simulink model "Pedal_Interpretation_exe"  (Simulink 7.0)
settings: Solver=ode4  StartTime=0.0  StopTime=88  FixedStep=0.01  RelTol=1e-3
InitFcn:
  | PedalInterp_para
values from neighbouring files (symbols this model uses):
  ped_min = 5    [PedalInterp_para.m]
  T_max_Brake = 4000    [PedalInterp_para.m]
  TI = 0    [PAS_callback.m]
undefined symbols (not defined in the file or in its folder): fzgbib, m_ab_100pro, m_ab_70pro, PedalInterpretation, v_bereich
libraries: simulink x320
(part 9 of 23)

== system Pedal_Interpretation_exe/TestData 1/SR-PI-02.2 Acceleration pedal interpretation/v = const & phi_Acc decreases & T_des_Drive < 0/Generate decrease 7/Generate  limited decrease for partition1 variant2 1 ==
  Repeating Sequence : Subsystem  mask(Repeating table){rep_seq_t=[0 T], rep_seq_y=[X0 XF]}
      mask prompts: rep_seq_t "Time values:"; rep_seq_y "Output values:"
      mask help: Output a repeating sequence of numbers specified in a table of time-value pairs. Values of time should be monotonically increasing.
      mask init: same as Pedal_Interpretation_exe/TestData 1/SR-PI-01.1 Brake Pedal recognition/phi_Brake < ped_min/Generate decrease 2/Generate  limited decrease for partition1 variant1 1/Repeating Sequence
      mask Help: Repeats cycle given in table. Time values should be monotonically increasing.
      mask Display: plot( disp_seq_t, disp_seq_y )
  Out1 : Outport  OutDataType=sfix(16)  OutScaling=2^0
  wires:
  Repeating Sequence/1(Out1) -> Out1/1

== system Pedal_Interpretation_exe/TestData 1/SR-PI-02.2 Acceleration pedal interpretation/v = const & phi_Acc decreases & T_des_Drive < 0/Generate decrease 7/TestDataVariants Sequence ==
  Constant : Constant  Value=2  OutDataType=sfix(16)  OutScaling=2^0
  Relational Operator : RelationalOperator  Operator=<=  LogicOutDataTypeMode=boolean
  Switch : Switch  Criteria=u2 ~= 0  OutDataType=sfix(16)  OutScaling=2^0
  Out1 : Outport  OutDataType=sfix(16)  OutScaling=2^0
  wires:
  [A] -> Relational Operator/1, Switch/1
  Constant/1 -> Relational Operator/2, Switch/3
  Relational Operator/1 -> Switch/2
  Switch/1 -> Out1/1

== system Pedal_Interpretation_exe/TestData 1/SR-PI-02.2 Acceleration pedal interpretation/v = const & phi_Acc decreases & T_des_Drive >= 0/Generate constant 6/Generate  constant for partition1 variant1 1 ==
  Repeating Sequence : Subsystem  mask(Repeating table){rep_seq_t=[0 T], rep_seq_y=[X0 X0]}
      mask prompts: rep_seq_t "Time values:"; rep_seq_y "Output values:"
      mask help: Output a repeating sequence of numbers specified in a table of time-value pairs. Values of time should be monotonically increasing.
      mask init: same as Pedal_Interpretation_exe/TestData 1/SR-PI-01.1 Brake Pedal recognition/phi_Brake < ped_min/Generate decrease 2/Generate  limited decrease for partition1 variant1 1/Repeating Sequence
      mask Help: Repeats cycle given in table. Time values should be monotonically increasing.
      mask Display: plot( disp_seq_t, disp_seq_y )
  Out1 : Outport  OutDataType=sfix(16)  OutScaling=2^0
  wires:
  Repeating Sequence/1(Out1) -> Out1/1

== system Pedal_Interpretation_exe/TestData 1/SR-PI-02.2 Acceleration pedal interpretation/v = const & phi_Acc decreases & T_des_Drive >= 0/Generate constant 6/Generate  constant for partition1 variant2 1 ==
  Repeating Sequence : Subsystem  mask(Repeating table){rep_seq_t=[0 T], rep_seq_y=[X0 X0]}
      mask prompts: rep_seq_t "Time values:"; rep_seq_y "Output values:"
      mask help: Output a repeating sequence of numbers specified in a table of time-value pairs. Values of time should be monotonically increasing.
      mask init: same as Pedal_Interpretation_exe/TestData 1/SR-PI-01.1 Brake Pedal recognition/phi_Brake < ped_min/Generate decrease 2/Generate  limited decrease for partition1 variant1 1/Repeating Sequence
      mask Help: Repeats cycle given in table. Time values should be monotonically increasing.
      mask Display: plot( disp_seq_t, disp_seq_y )
  Out1 : Outport  OutDataType=sfix(16)  OutScaling=2^0
  wires:
  Repeating Sequence/1(Out1) -> Out1/1

== system Pedal_Interpretation_exe/TestData 1/SR-PI-02.2 Acceleration pedal interpretation/v = const & phi_Acc decreases & T_des_Drive >= 0/Generate constant 6/Generate  constant for partition1 variant3 1 ==
  Repeating Sequence : Subsystem  mask(Repeating table){rep_seq_t=[0 T], rep_seq_y=[X0 X0]}
      mask prompts: rep_seq_t "Time values:"; rep_seq_y "Output values:"
      mask help: Output a repeating sequence of numbers specified in a table of time-value pairs. Values of time should be monotonically increasing.
      mask init: same as Pedal_Interpretation_exe/TestData 1/SR-PI-01.1 Brake Pedal recognition/phi_Brake < ped_min/Generate decrease 2/Generate  limited decrease for partition1 variant1 1/Repeating Sequence
      mask Help: Repeats cycle given in table. Time values should be monotonically increasing.
      mask Display: plot( disp_seq_t, disp_seq_y )
  Out1 : Outport  OutDataType=sfix(16)  OutScaling=2^0
  wires:
  Repeating Sequence/1(Out1) -> Out1/1

== system Pedal_Interpretation_exe/TestData 1/SR-PI-02.2 Acceleration pedal interpretation/v = const & phi_Acc decreases & T_des_Drive >= 0/Generate constant 6/Generate  constant for partition1 variant4 1 ==
  Repeating Sequence : Subsystem  mask(Repeating table){rep_seq_t=[0 T], rep_seq_y=[X0 X0]}
      mask prompts: rep_seq_t "Time values:"; rep_seq_y "Output values:"
      mask help: Output a repeating sequence of numbers specified in a table of time-value pairs. Values of time should be monotonically increasing.
      mask init: same as Pedal_Interpretation_exe/TestData 1/SR-PI-01.1 Brake Pedal recognition/phi_Brake < ped_min/Generate decrease 2/Generate  limited decrease for partition1 variant1 1/Repeating Sequence
      mask Help: Repeats cycle given in table. Time values should be monotonically increasing.
      mask Display: plot( disp_seq_t, disp_seq_y )
  Out1 : Outport  OutDataType=sfix(16)  OutScaling=2^0
  wires:
  Repeating Sequence/1(Out1) -> Out1/1

== system Pedal_Interpretation_exe/TestData 1/SR-PI-02.2 Acceleration pedal interpretation/v = const & phi_Acc decreases & T_des_Drive >= 0/Generate constant 6/Generate  constant for partition1 variant5 1 ==
  Repeating Sequence : Subsystem  mask(Repeating table){rep_seq_t=[0 T], rep_seq_y=[X0 X0]}
      mask prompts: rep_seq_t "Time values:"; rep_seq_y "Output values:"
      mask help: Output a repeating sequence of numbers specified in a table of time-value pairs. Values of time should be monotonically increasing.
      mask init: same as Pedal_Interpretation_exe/TestData 1/SR-PI-01.1 Brake Pedal recognition/phi_Brake < ped_min/Generate decrease 2/Generate  limited decrease for partition1 variant1 1/Repeating Sequence
      mask Help: Repeats cycle given in table. Time values should be monotonically increasing.
      mask Display: plot( disp_seq_t, disp_seq_y )
  Out1 : Outport  OutDataType=sfix(16)  OutScaling=2^0
  wires:
  Repeating Sequence/1(Out1) -> Out1/1

== system Pedal_Interpretation_exe/TestData 1/SR-PI-02.2 Acceleration pedal interpretation/v = const & phi_Acc decreases & T_des_Drive >= 0/Generate constant 6/TestDataVariants Sequence ==
  Constant : Constant  Value=5  OutDataType=sfix(16)  OutScaling=2^0
  Relational Operator : RelationalOperator  Operator=<=  LogicOutDataTypeMode=boolean
  Switch : Switch  Criteria=u2 ~= 0  OutDataType=sfix(16)  OutScaling=2^0
  Out1 : Outport  OutDataType=sfix(16)  OutScaling=2^0
  wires:
  [A] -> Relational Operator/1, Switch/1
  Constant/1 -> Relational Operator/2, Switch/3
  Relational Operator/1 -> Switch/2
  Switch/1 -> Out1/1

== system Pedal_Interpretation_exe/TestData 1/SR-PI-02.2 Acceleration pedal interpretation/v = const & phi_Acc decreases & T_des_Drive >= 0/Generate decrease 7/Generate  limited decrease for partition1 variant1 1 ==
  Repeating Sequence : Subsystem  mask(Repeating table){rep_seq_t=[0 T], rep_seq_y=[X0 XF]}
      mask prompts: rep_seq_t "Time values:"; rep_seq_y "Output values:"
      mask help: Output a repeating sequence of numbers specified in a table of time-value pairs. Values of time should be monotonically increasing.
      mask init: same as Pedal_Interpretation_exe/TestData 1/SR-PI-01.1 Brake Pedal recognition/phi_Brake < ped_min/Generate decrease 2/Generate  limited decrease for partition1 variant1 1/Repeating Sequence
      mask Help: Repeats cycle given in table. Time values should be monotonically increasing.
      mask Display: plot( disp_seq_t, disp_seq_y )
  Out1 : Outport  OutDataType=sfix(16)  OutScaling=2^0
  wires:
  Repeating Sequence/1(Out1) -> Out1/1

== system Pedal_Interpretation_exe/TestData 1/SR-PI-02.2 Acceleration pedal interpretation/v = const & phi_Acc decreases & T_des_Drive >= 0/Generate decrease 7/Generate  limited decrease for partition1 variant2 1 ==
  Repeating Sequence : Subsystem  mask(Repeating table){rep_seq_t=[0 T], rep_seq_y=[X0 XF]}
      mask prompts: rep_seq_t "Time values:"; rep_seq_y "Output values:"
      mask help: Output a repeating sequence of numbers specified in a table of time-value pairs. Values of time should be monotonically increasing.
      mask init: same as Pedal_Interpretation_exe/TestData 1/SR-PI-01.1 Brake Pedal recognition/phi_Brake < ped_min/Generate decrease 2/Generate  limited decrease for partition1 variant1 1/Repeating Sequence
      mask Help: Repeats cycle given in table. Time values should be monotonically increasing.
      mask Display: plot( disp_seq_t, disp_seq_y )
  Out1 : Outport  OutDataType=sfix(16)  OutScaling=2^0
  wires:
  Repeating Sequence/1(Out1) -> Out1/1

== system Pedal_Interpretation_exe/TestData 1/SR-PI-02.2 Acceleration pedal interpretation/v = const & phi_Acc decreases & T_des_Drive >= 0/Generate decrease 7/TestDataVariants Sequence ==
  Constant : Constant  Value=2  OutDataType=sfix(16)  OutScaling=2^0
  Relational Operator : RelationalOperator  Operator=<=  LogicOutDataTypeMode=boolean
  Switch : Switch  Criteria=u2 ~= 0  OutDataType=sfix(16)  OutScaling=2^0
  Out1 : Outport  OutDataType=sfix(16)  OutScaling=2^0
  wires:
  [A] -> Relational Operator/1, Switch/1
  Constant/1 -> Relational Operator/2, Switch/3
  Relational Operator/1 -> Switch/2
  Switch/1 -> Out1/1

== system Pedal_Interpretation_exe/TestData 1/SR-PI-02.2 Acceleration pedal interpretation/v = const & phi_Acc increases & T_des_Drive < 0/Generate constant 6/Generate  constant for partition1 variant1 1 ==
  Repeating Sequence : Subsystem  mask(Repeating table){rep_seq_t=[0 T], rep_seq_y=[X0 X0]}
      mask prompts: rep_seq_t "Time values:"; rep_seq_y "Output values:"
      mask help: Output a repeating sequence of numbers specified in a table of time-value pairs. Values of time should be monotonically increasing.
      mask init: same as Pedal_Interpretation_exe/TestData 1/SR-PI-01.1 Brake Pedal recognition/phi_Brake < ped_min/Generate decrease 2/Generate  limited decrease for partition1 variant1 1/Repeating Sequence
      mask Help: Repeats cycle given in table. Time values should be monotonically increasing.
      mask Display: plot( disp_seq_t, disp_seq_y )
  Out1 : Outport  OutDataType=sfix(16)  OutScaling=2^0
  wires:
  Repeating Sequence/1(Out1) -> Out1/1

== system Pedal_Interpretation_exe/TestData 1/SR-PI-02.2 Acceleration pedal interpretation/v = const & phi_Acc increases & T_des_Drive < 0/Generate constant 6/Generate  constant for partition1 variant2 1 ==
  Repeating Sequence : Subsystem  mask(Repeating table){rep_seq_t=[0 T], rep_seq_y=[X0 X0]}
      mask prompts: rep_seq_t "Time values:"; rep_seq_y "Output values:"
      mask help: Output a repeating sequence of numbers specified in a table of time-value pairs. Values of time should be monotonically increasing.
      mask init: same as Pedal_Interpretation_exe/TestData 1/SR-PI-01.1 Brake Pedal recognition/phi_Brake < ped_min/Generate decrease 2/Generate  limited decrease for partition1 variant1 1/Repeating Sequence
      mask Help: Repeats cycle given in table. Time values should be monotonically increasing.
      mask Display: plot( disp_seq_t, disp_seq_y )
  Out1 : Outport  OutDataType=sfix(16)  OutScaling=2^0
  wires:
  Repeating Sequence/1(Out1) -> Out1/1

== system Pedal_Interpretation_exe/TestData 1/SR-PI-02.2 Acceleration pedal interpretation/v = const & phi_Acc increases & T_des_Drive < 0/Generate constant 6/Generate  constant for partition1 variant3 1 ==
  Repeating Sequence : Subsystem  mask(Repeating table){rep_seq_t=[0 T], rep_seq_y=[X0 X0]}
      mask prompts: rep_seq_t "Time values:"; rep_seq_y "Output values:"
      mask help: Output a repeating sequence of numbers specified in a table of time-value pairs. Values of time should be monotonically increasing.
      mask init: same as Pedal_Interpretation_exe/TestData 1/SR-PI-01.1 Brake Pedal recognition/phi_Brake < ped_min/Generate decrease 2/Generate  limited decrease for partition1 variant1 1/Repeating Sequence
      mask Help: Repeats cycle given in table. Time values should be monotonically increasing.
      mask Display: plot( disp_seq_t, disp_seq_y )
  Out1 : Outport  OutDataType=sfix(16)  OutScaling=2^0
  wires:
  Repeating Sequence/1(Out1) -> Out1/1

== system Pedal_Interpretation_exe/TestData 1/SR-PI-02.2 Acceleration pedal interpretation/v = const & phi_Acc increases & T_des_Drive < 0/Generate constant 6/Generate  constant for partition1 variant4 1 ==
  Repeating Sequence : Subsystem  mask(Repeating table){rep_seq_t=[0 T], rep_seq_y=[X0 X0]}
      mask prompts: rep_seq_t "Time values:"; rep_seq_y "Output values:"
      mask help: Output a repeating sequence of numbers specified in a table of time-value pairs. Values of time should be monotonically increasing.
      mask init: same as Pedal_Interpretation_exe/TestData 1/SR-PI-01.1 Brake Pedal recognition/phi_Brake < ped_min/Generate decrease 2/Generate  limited decrease for partition1 variant1 1/Repeating Sequence
      mask Help: Repeats cycle given in table. Time values should be monotonically increasing.
      mask Display: plot( disp_seq_t, disp_seq_y )
  Out1 : Outport  OutDataType=sfix(16)  OutScaling=2^0
  wires:
  Repeating Sequence/1(Out1) -> Out1/1

== system Pedal_Interpretation_exe/TestData 1/SR-PI-02.2 Acceleration pedal interpretation/v = const & phi_Acc increases & T_des_Drive < 0/Generate constant 6/Generate  constant for partition1 variant5 1 ==
  Repeating Sequence : Subsystem  mask(Repeating table){rep_seq_t=[0 T], rep_seq_y=[X0 X0]}
      mask prompts: rep_seq_t "Time values:"; rep_seq_y "Output values:"
      mask help: Output a repeating sequence of numbers specified in a table of time-value pairs. Values of time should be monotonically increasing.
      mask init: same as Pedal_Interpretation_exe/TestData 1/SR-PI-01.1 Brake Pedal recognition/phi_Brake < ped_min/Generate decrease 2/Generate  limited decrease for partition1 variant1 1/Repeating Sequence
      mask Help: Repeats cycle given in table. Time values should be monotonically increasing.
      mask Display: plot( disp_seq_t, disp_seq_y )
  Out1 : Outport  OutDataType=sfix(16)  OutScaling=2^0
  wires:
  Repeating Sequence/1(Out1) -> Out1/1

== system Pedal_Interpretation_exe/TestData 1/SR-PI-02.2 Acceleration pedal interpretation/v = const & phi_Acc increases & T_des_Drive < 0/Generate constant 6/TestDataVariants Sequence ==
  Constant : Constant  Value=5  OutDataType=sfix(16)  OutScaling=2^0
  Relational Operator : RelationalOperator  Operator=<=  LogicOutDataTypeMode=boolean
  Switch : Switch  Criteria=u2 ~= 0  OutDataType=sfix(16)  OutScaling=2^0
  Out1 : Outport  OutDataType=sfix(16)  OutScaling=2^0
  wires:
  [A] -> Relational Operator/1, Switch/1
  Constant/1 -> Relational Operator/2, Switch/3
  Relational Operator/1 -> Switch/2
  Switch/1 -> Out1/1

== system Pedal_Interpretation_exe/TestData 1/SR-PI-02.2 Acceleration pedal interpretation/v = const & phi_Acc increases & T_des_Drive < 0/Generate increase 7/Generate  limited increase for partition1 variant1 1 ==
  Repeating Sequence : Subsystem  mask(Repeating table){rep_seq_t=[0 T], rep_seq_y=[X0 XF]}
      mask prompts: rep_seq_t "Time values:"; rep_seq_y "Output values:"
      mask help: Output a repeating sequence of numbers specified in a table of time-value pairs. Values of time should be monotonically increasing.
      mask init: same as Pedal_Interpretation_exe/TestData 1/SR-PI-01.1 Brake Pedal recognition/phi_Brake < ped_min/Generate decrease 2/Generate  limited decrease for partition1 variant1 1/Repeating Sequence
      mask Help: Repeats cycle given in table. Time values should be monotonically increasing.
      mask Display: plot( disp_seq_t, disp_seq_y )
  Out1 : Outport  OutDataType=sfix(16)  OutScaling=2^0
  wires:
  Repeating Sequence/1(Out1) -> Out1/1

== system Pedal_Interpretation_exe/TestData 1/SR-PI-02.2 Acceleration pedal interpretation/v = const & phi_Acc increases & T_des_Drive < 0/Generate increase 7/Generate  limited increase for partition1 variant2 1 ==
  Repeating Sequence : Subsystem  mask(Repeating table){rep_seq_t=[0 T], rep_seq_y=[X0 XF]}
      mask prompts: rep_seq_t "Time values:"; rep_seq_y "Output values:"
      mask help: Output a repeating sequence of numbers specified in a table of time-value pairs. Values of time should be monotonically increasing.
      mask init: same as Pedal_Interpretation_exe/TestData 1/SR-PI-01.1 Brake Pedal recognition/phi_Brake < ped_min/Generate decrease 2/Generate  limited decrease for partition1 variant1 1/Repeating Sequence
      mask Help: Repeats cycle given in table. Time values should be monotonically increasing.
      mask Display: plot( disp_seq_t, disp_seq_y )
  Out1 : Outport  OutDataType=sfix(16)  OutScaling=2^0
  wires:
  Repeating Sequence/1(Out1) -> Out1/1

== system Pedal_Interpretation_exe/TestData 1/SR-PI-02.2 Acceleration pedal interpretation/v = const & phi_Acc increases & T_des_Drive < 0/Generate increase 7/TestDataVariants Sequence ==
  Constant : Constant  Value=2  OutDataType=sfix(16)  OutScaling=2^0
  Relational Operator : RelationalOperator  Operator=<=  LogicOutDataTypeMode=boolean
  Switch : Switch  Criteria=u2 ~= 0  OutDataType=sfix(16)  OutScaling=2^0
  Out1 : Outport  OutDataType=sfix(16)  OutScaling=2^0
  wires:
  [A] -> Relational Operator/1, Switch/1
  Constant/1 -> Relational Operator/2, Switch/3
  Relational Operator/1 -> Switch/2
  Switch/1 -> Out1/1

== system Pedal_Interpretation_exe/TestData 1/SR-PI-02.2 Acceleration pedal interpretation/v = const & phi_Acc increases & T_des_Drive >= 0/Generate constant 6/Generate  constant for partition1 variant1 1 ==
  Repeating Sequence : Subsystem  mask(Repeating table){rep_seq_t=[0 T], rep_seq_y=[X0 X0]}
      mask prompts: rep_seq_t "Time values:"; rep_seq_y "Output values:"
      mask help: Output a repeating sequence of numbers specified in a table of time-value pairs. Values of time should be monotonically increasing.
      mask init: same as Pedal_Interpretation_exe/TestData 1/SR-PI-01.1 Brake Pedal recognition/phi_Brake < ped_min/Generate decrease 2/Generate  limited decrease for partition1 variant1 1/Repeating Sequence
      mask Help: Repeats cycle given in table. Time values should be monotonically increasing.
      mask Display: plot( disp_seq_t, disp_seq_y )
  Out1 : Outport  OutDataType=sfix(16)  OutScaling=2^0
  wires:
  Repeating Sequence/1(Out1) -> Out1/1

== system Pedal_Interpretation_exe/TestData 1/SR-PI-02.2 Acceleration pedal interpretation/v = const & phi_Acc increases & T_des_Drive >= 0/Generate constant 6/Generate  constant for partition1 variant2 1 ==
  Repeating Sequence : Subsystem  mask(Repeating table){rep_seq_t=[0 T], rep_seq_y=[X0 X0]}
      mask prompts: rep_seq_t "Time values:"; rep_seq_y "Output values:"
      mask help: Output a repeating sequence of numbers specified in a table of time-value pairs. Values of time should be monotonically increasing.
      mask init: same as Pedal_Interpretation_exe/TestData 1/SR-PI-01.1 Brake Pedal recognition/phi_Brake < ped_min/Generate decrease 2/Generate  limited decrease for partition1 variant1 1/Repeating Sequence
      mask Help: Repeats cycle given in table. Time values should be monotonically increasing.
      mask Display: plot( disp_seq_t, disp_seq_y )
  Out1 : Outport  OutDataType=sfix(16)  OutScaling=2^0
  wires:
  Repeating Sequence/1(Out1) -> Out1/1

== system Pedal_Interpretation_exe/TestData 1/SR-PI-02.2 Acceleration pedal interpretation/v = const & phi_Acc increases & T_des_Drive >= 0/Generate constant 6/Generate  constant for partition1 variant3 1 ==
  Repeating Sequence : Subsystem  mask(Repeating table){rep_seq_t=[0 T], rep_seq_y=[X0 X0]}
      mask prompts: rep_seq_t "Time values:"; rep_seq_y "Output values:"
      mask help: Output a repeating sequence of numbers specified in a table of time-value pairs. Values of time should be monotonically increasing.
      mask init: same as Pedal_Interpretation_exe/TestData 1/SR-PI-01.1 Brake Pedal recognition/phi_Brake < ped_min/Generate decrease 2/Generate  limited decrease for partition1 variant1 1/Repeating Sequence
      mask Help: Repeats cycle given in table. Time values should be monotonically increasing.
      mask Display: plot( disp_seq_t, disp_seq_y )
  Out1 : Outport  OutDataType=sfix(16)  OutScaling=2^0
  wires:
  Repeating Sequence/1(Out1) -> Out1/1

== system Pedal_Interpretation_exe/TestData 1/SR-PI-02.2 Acceleration pedal interpretation/v = const & phi_Acc increases & T_des_Drive >= 0/Generate constant 6/Generate  constant for partition1 variant4 1 ==
  Repeating Sequence : Subsystem  mask(Repeating table){rep_seq_t=[0 T], rep_seq_y=[X0 X0]}
      mask prompts: rep_seq_t "Time values:"; rep_seq_y "Output values:"
      mask help: Output a repeating sequence of numbers specified in a table of time-value pairs. Values of time should be monotonically increasing.
      mask init: same as Pedal_Interpretation_exe/TestData 1/SR-PI-01.1 Brake Pedal recognition/phi_Brake < ped_min/Generate decrease 2/Generate  limited decrease for partition1 variant1 1/Repeating Sequence
      mask Help: Repeats cycle given in table. Time values should be monotonically increasing.
      mask Display: plot( disp_seq_t, disp_seq_y )
  Out1 : Outport  OutDataType=sfix(16)  OutScaling=2^0
  wires:
  Repeating Sequence/1(Out1) -> Out1/1

== system Pedal_Interpretation_exe/TestData 1/SR-PI-02.2 Acceleration pedal interpretation/v = const & phi_Acc increases & T_des_Drive >= 0/Generate constant 6/Generate  constant for partition1 variant5 1 ==
  Repeating Sequence : Subsystem  mask(Repeating table){rep_seq_t=[0 T], rep_seq_y=[X0 X0]}
      mask prompts: rep_seq_t "Time values:"; rep_seq_y "Output values:"
      mask help: Output a repeating sequence of numbers specified in a table of time-value pairs. Values of time should be monotonically increasing.
      mask init: same as Pedal_Interpretation_exe/TestData 1/SR-PI-01.1 Brake Pedal recognition/phi_Brake < ped_min/Generate decrease 2/Generate  limited decrease for partition1 variant1 1/Repeating Sequence
      mask Help: Repeats cycle given in table. Time values should be monotonically increasing.
      mask Display: plot( disp_seq_t, disp_seq_y )
  Out1 : Outport  OutDataType=sfix(16)  OutScaling=2^0
  wires:
  Repeating Sequence/1(Out1) -> Out1/1

== system Pedal_Interpretation_exe/TestData 1/SR-PI-02.2 Acceleration pedal interpretation/v = const & phi_Acc increases & T_des_Drive >= 0/Generate constant 6/TestDataVariants Sequence ==
  Constant : Constant  Value=5  OutDataType=sfix(16)  OutScaling=2^0
  Relational Operator : RelationalOperator  Operator=<=  LogicOutDataTypeMode=boolean
  Switch : Switch  Criteria=u2 ~= 0  OutDataType=sfix(16)  OutScaling=2^0
  Out1 : Outport  OutDataType=sfix(16)  OutScaling=2^0
  wires:
  [A] -> Relational Operator/1, Switch/1
  Constant/1 -> Relational Operator/2, Switch/3
  Relational Operator/1 -> Switch/2
  Switch/1 -> Out1/1

== system Pedal_Interpretation_exe/TestData 1/SR-PI-02.2 Acceleration pedal interpretation/v = const & phi_Acc increases & T_des_Drive >= 0/Generate increase 7/Generate  limited increase for partition1 variant1 1 ==
  Repeating Sequence : Subsystem  mask(Repeating table){rep_seq_t=[0 T], rep_seq_y=[X0 XF]}
      mask prompts: rep_seq_t "Time values:"; rep_seq_y "Output values:"
      mask help: Output a repeating sequence of numbers specified in a table of time-value pairs. Values of time should be monotonically increasing.
      mask init: same as Pedal_Interpretation_exe/TestData 1/SR-PI-01.1 Brake Pedal recognition/phi_Brake < ped_min/Generate decrease 2/Generate  limited decrease for partition1 variant1 1/Repeating Sequence
      mask Help: Repeats cycle given in table. Time values should be monotonically increasing.
      mask Display: plot( disp_seq_t, disp_seq_y )
  Out1 : Outport  OutDataType=sfix(16)  OutScaling=2^0
  wires:
  Repeating Sequence/1(Out1) -> Out1/1

== system Pedal_Interpretation_exe/TestData 1/SR-PI-02.2 Acceleration pedal interpretation/v = const & phi_Acc increases & T_des_Drive >= 0/Generate increase 7/Generate  limited increase for partition1 variant2 1 ==
  Repeating Sequence : Subsystem  mask(Repeating table){rep_seq_t=[0 T], rep_seq_y=[X0 XF]}
      mask prompts: rep_seq_t "Time values:"; rep_seq_y "Output values:"
      mask help: Output a repeating sequence of numbers specified in a table of time-value pairs. Values of time should be monotonically increasing.
      mask init: same as Pedal_Interpretation_exe/TestData 1/SR-PI-01.1 Brake Pedal recognition/phi_Brake < ped_min/Generate decrease 2/Generate  limited decrease for partition1 variant1 1/Repeating Sequence
      mask Help: Repeats cycle given in table. Time values should be monotonically increasing.
      mask Display: plot( disp_seq_t, disp_seq_y )
  Out1 : Outport  OutDataType=sfix(16)  OutScaling=2^0
  wires:
  Repeating Sequence/1(Out1) -> Out1/1

== system Pedal_Interpretation_exe/TestData 1/SR-PI-02.2 Acceleration pedal interpretation/v = const & phi_Acc increases & T_des_Drive >= 0/Generate increase 7/TestDataVariants Sequence ==
  Constant : Constant  Value=2  OutDataType=sfix(16)  OutScaling=2^0
  Relational Operator : RelationalOperator  Operator=<=  LogicOutDataTypeMode=boolean
  Switch : Switch  Criteria=u2 ~= 0  OutDataType=sfix(16)  OutScaling=2^0
  Out1 : Outport  OutDataType=sfix(16)  OutScaling=2^0
  wires:
  [A] -> Relational Operator/1, Switch/1
  Constant/1 -> Relational Operator/2, Switch/3
  Relational Operator/1 -> Switch/2
  Switch/1 -> Out1/1

== system Pedal_Interpretation_exe/TestData 1/SR-PI-02.2 Acceleration pedal interpretation/v increases & phi_Acc = const & T_des_Drive >= 0/Generate constant 6/Generate  constant for partition1 variant1 1 ==
  Repeating Sequence : Subsystem  mask(Repeating table){rep_seq_t=[0 T], rep_seq_y=[X0 X0]}
      mask prompts: rep_seq_t "Time values:"; rep_seq_y "Output values:"
      mask help: Output a repeating sequence of numbers specified in a table of time-value pairs. Values of time should be monotonically increasing.
      mask init: same as Pedal_Interpretation_exe/TestData 1/SR-PI-01.1 Brake Pedal recognition/phi_Brake < ped_min/Generate decrease 2/Generate  limited decrease for partition1 variant1 1/Repeating Sequence
      mask Help: Repeats cycle given in table. Time values should be monotonically increasing.
      mask Display: plot( disp_seq_t, disp_seq_y )
  Out1 : Outport  OutDataType=sfix(16)  OutScaling=2^0
  wires:
  Repeating Sequence/1(Out1) -> Out1/1

== system Pedal_Interpretation_exe/TestData 1/SR-PI-02.2 Acceleration pedal interpretation/v increases & phi_Acc = const & T_des_Drive >= 0/Generate constant 6/Generate  constant for partition1 variant2 1 ==
  Repeating Sequence : Subsystem  mask(Repeating table){rep_seq_t=[0 T], rep_seq_y=[X0 X0]}
      mask prompts: rep_seq_t "Time values:"; rep_seq_y "Output values:"
      mask help: Output a repeating sequence of numbers specified in a table of time-value pairs. Values of time should be monotonically increasing.
      mask init: same as Pedal_Interpretation_exe/TestData 1/SR-PI-01.1 Brake Pedal recognition/phi_Brake < ped_min/Generate decrease 2/Generate  limited decrease for partition1 variant1 1/Repeating Sequence
      mask Help: Repeats cycle given in table. Time values should be monotonically increasing.
      mask Display: plot( disp_seq_t, disp_seq_y )
  Out1 : Outport  OutDataType=sfix(16)  OutScaling=2^0
  wires:
  Repeating Sequence/1(Out1) -> Out1/1

== system Pedal_Interpretation_exe/TestData 1/SR-PI-02.2 Acceleration pedal interpretation/v increases & phi_Acc = const & T_des_Drive >= 0/Generate constant 6/Generate  constant for partition1 variant3 1 ==
  Repeating Sequence : Subsystem  mask(Repeating table){rep_seq_t=[0 T], rep_seq_y=[X0 X0]}
      mask prompts: rep_seq_t "Time values:"; rep_seq_y "Output values:"
      mask help: Output a repeating sequence of numbers specified in a table of time-value pairs. Values of time should be monotonically increasing.
      mask init: same as Pedal_Interpretation_exe/TestData 1/SR-PI-01.1 Brake Pedal recognition/phi_Brake < ped_min/Generate decrease 2/Generate  limited decrease for partition1 variant1 1/Repeating Sequence
      mask Help: Repeats cycle given in table. Time values should be monotonically increasing.
      mask Display: plot( disp_seq_t, disp_seq_y )
  Out1 : Outport  OutDataType=sfix(16)  OutScaling=2^0
  wires:
  Repeating Sequence/1(Out1) -> Out1/1

== system Pedal_Interpretation_exe/TestData 1/SR-PI-02.2 Acceleration pedal interpretation/v increases & phi_Acc = const & T_des_Drive >= 0/Generate constant 6/TestDataVariants Sequence ==
  Constant : Constant  Value=3  OutDataType=sfix(16)  OutScaling=2^0
  Relational Operator : RelationalOperator  Operator=<=  LogicOutDataTypeMode=boolean
  Switch : Switch  Criteria=u2 ~= 0  OutDataType=sfix(16)  OutScaling=2^0
  Out1 : Outport  OutDataType=sfix(16)  OutScaling=2^0
  wires:
  [A] -> Relational Operator/1, Switch/1
  Constant/1 -> Relational Operator/2, Switch/3
  Relational Operator/1 -> Switch/2
  Switch/1 -> Out1/1

== system Pedal_Interpretation_exe/TestData 1/SR-PI-02.2 Acceleration pedal interpretation/v increases & phi_Acc = const & T_des_Drive >= 0/Generate increase 7/Generate  limited increase for partition1 variant1 1 ==
  Repeating Sequence : Subsystem  mask(Repeating table){rep_seq_t=[0 T], rep_seq_y=[X0 XF]}
      mask prompts: rep_seq_t "Time values:"; rep_seq_y "Output values:"
      mask help: Output a repeating sequence of numbers specified in a table of time-value pairs. Values of time should be monotonically increasing.
      mask init: same as Pedal_Interpretation_exe/TestData 1/SR-PI-01.1 Brake Pedal recognition/phi_Brake < ped_min/Generate decrease 2/Generate  limited decrease for partition1 variant1 1/Repeating Sequence
      mask Help: Repeats cycle given in table. Time values should be monotonically increasing.
      mask Display: plot( disp_seq_t, disp_seq_y )
  Out1 : Outport  OutDataType=sfix(16)  OutScaling=2^0
  wires:
  Repeating Sequence/1(Out1) -> Out1/1

== system Pedal_Interpretation_exe/TestData 1/SR-PI-02.2 Acceleration pedal interpretation/v increases & phi_Acc = const & T_des_Drive >= 0/Generate increase 7/Generate  limited increase for partition1 variant2 1 ==
  Repeating Sequence : Subsystem  mask(Repeating table){rep_seq_t=[0 T], rep_seq_y=[X0 XF]}
      mask prompts: rep_seq_t "Time values:"; rep_seq_y "Output values:"
      mask help: Output a repeating sequence of numbers specified in a table of time-value pairs. Values of time should be monotonically increasing.
      mask init: same as Pedal_Interpretation_exe/TestData 1/SR-PI-01.1 Brake Pedal recognition/phi_Brake < ped_min/Generate decrease 2/Generate  limited decrease for partition1 variant1 1/Repeating Sequence
      mask Help: Repeats cycle given in table. Time values should be monotonically increasing.
      mask Display: plot( disp_seq_t, disp_seq_y )
  Out1 : Outport  OutDataType=sfix(16)  OutScaling=2^0
  wires:
  Repeating Sequence/1(Out1) -> Out1/1

== system Pedal_Interpretation_exe/TestData 1/SR-PI-02.2 Acceleration pedal interpretation/v increases & phi_Acc = const & T_des_Drive >= 0/Generate increase 7/Generate  limited increase for partition2 variant1 1 ==
  Repeating Sequence : Subsystem  mask(Repeating table){rep_seq_t=[0 T], rep_seq_y=[X0 XF]}
      mask prompts: rep_seq_t "Time values:"; rep_seq_y "Output values:"
      mask help: Output a repeating sequence of numbers specified in a table of time-value pairs. Values of time should be monotonically increasing.
      mask init: same as Pedal_Interpretation_exe/TestData 1/SR-PI-01.1 Brake Pedal recognition/phi_Brake < ped_min/Generate decrease 2/Generate  limited decrease for partition1 variant1 1/Repeating Sequence
      mask Help: Repeats cycle given in table. Time values should be monotonically increasing.
      mask Display: plot( disp_seq_t, disp_seq_y )
  Out1 : Outport  OutDataType=sfix(16)  OutScaling=2^0
  wires:
  Repeating Sequence/1(Out1) -> Out1/1

== system Pedal_Interpretation_exe/TestData 1/SR-PI-02.2 Acceleration pedal interpretation/v increases & phi_Acc = const & T_des_Drive >= 0/Generate increase 7/Generate  limited increase for partition2 variant2 1 ==
  Repeating Sequence : Subsystem  mask(Repeating table){rep_seq_t=[0 T], rep_seq_y=[X0 XF]}
      mask prompts: rep_seq_t "Time values:"; rep_seq_y "Output values:"
      mask help: Output a repeating sequence of numbers specified in a table of time-value pairs. Values of time should be monotonically increasing.
      mask init: same as Pedal_Interpretation_exe/TestData 1/SR-PI-01.1 Brake Pedal recognition/phi_Brake < ped_min/Generate decrease 2/Generate  limited decrease for partition1 variant1 1/Repeating Sequence
      mask Help: Repeats cycle given in table. Time values should be monotonically increasing.
      mask Display: plot( disp_seq_t, disp_seq_y )
  Out1 : Outport  OutDataType=sfix(16)  OutScaling=2^0
  wires:
  Repeating Sequence/1(Out1) -> Out1/1

== system Pedal_Interpretation_exe/TestData 1/SR-PI-02.2 Acceleration pedal interpretation/v increases & phi_Acc = const & T_des_Drive >= 0/Generate increase 7/TestDataVariants Sequence ==
  Constant : Constant  Value=4  OutDataType=sfix(16)  OutScaling=2^0
  Relational Operator : RelationalOperator  Operator=<=  LogicOutDataTypeMode=boolean
  Switch : Switch  Criteria=u2 ~= 0  OutDataType=sfix(16)  OutScaling=2^0
  Out1 : Outport  OutDataType=sfix(16)  OutScaling=2^0
  wires:
  [A] -> Relational Operator/1, Switch/1
  Constant/1 -> Relational Operator/2, Switch/3
  Relational Operator/1 -> Switch/2
  Switch/1 -> Out1/1

== system Pedal_Interpretation_exe/Validation Functions/SR-PI-01.1 Brake Pedal recognition/BrakePedal == 0/PAS/A delay ==
  In1 : Inport  OutDataType=sfix(16)  OutScaling=2^0
  Data Type Conversion : DataTypeConversion  OutDataType=sfix(16)  OutScaling=2^0
  Delay : Constant  Value=0  OutDataType=sfix(16)  OutScaling=2^0
  Integer Delay : S-Function  FunctionName=sfix_udelay  Parameters=samptime,vinit,NumDelays,1,1,0  mask(Integer Delay){vinit=0.0, samptime=-1, NumDelays=600}
      mask prompts: vinit "Initial condition:"; samptime "Sample time:"; NumDelays "Number of delays:"
      mask help: Delay a signal N sample periods.
      mask init:
      | if isempty(NumDelays)
      |    NumDelays = 1;
      | end
      mask Display: fprintf(' %d\nZ   ',-1*(NumDelays))
  Switch : Switch  Criteria=u2 ~= 0
  Out1 : Outport  OutDataType=sfix(16)  OutScaling=2^0
  wires:
  Data Type Conversion/1 -> Out1/1
  Integer Delay/1 -> Switch/1
  Delay/1 -> Switch/2
  In1/1 -> Integer Delay/1, Switch/3
  Switch/1 -> Data Type Conversion/1

== system Pedal_Interpretation_exe/Validation Functions/SR-PI-01.1 Brake Pedal recognition/BrakePedal == 0/PAS/Delay bus signals ==
  ELLin : Inport  OutDataType=sfix(16)  OutScaling=2^0
  EULin : Inport  Port=2  OutDataType=sfix(16)  OutScaling=2^0
  ADin : Inport  Port=3  OutDataType=sfix(16)  OutScaling=2^0
  AD delay : Subsystem  TreatAsAtomicUnit=on  mask{Delay=0}
      mask prompts: Delay "Delay (in simulation steps) for the input signal:"
      mask init:
      | %set_param([gcb '/Discrete Transfer Fcn'],'Denominator',['[' num2str([1 zeros(1,str2double(get_param(gcb,'Delay')))]) ']']);
      mask CallbackString:
      | Delay = str2double(get_param(gcb,'Delay'));
      | if Delay < 0
      |     set_param(gcb,'Delay','0');
      |     error('Only non-negative delays are possible (causality).');
      |     set_param([gcb '/Delay'],'Value','0');
      | elseif Delay == 0
      |     set_param([gcb '/Delay'],'Value','0');
      | else
      |     set_param([gcb '/Integer Delay'],'NumDelays',num2str(Delay));
      |     set_param([gcb '/Delay'],'Value',num2str(Delay));
      | end
      mask Display: text(0.5,0.5,['z^{ ' num2str((-1)*str2double(get_param(gcb,'Delay'))) '}'],'texmode','on');
  ELL delay : Subsystem  TreatAsAtomicUnit=on  mask{Delay=0}
      mask prompts: Delay "Delay (in simulation steps) for the input signal:"
      mask init:
      | %set_param([gcb '/Discrete Transfer Fcn'],'Denominator',['[' num2str([1 zeros(1,str2double(get_param(gcb,'Delay')))]) ']']);
      mask CallbackString:
      | Delay = str2double(get_param(gcb,'Delay'));
      | if Delay < 0
      |     set_param(gcb,'Delay','0');
      |     error('Only non-negative delays are possible (causality).');
      |     set_param([gcb '/Delay'],'Value','0');
      | elseif Delay == 0
      |     set_param([gcb '/Delay'],'Value','0');
      | else
      |     set_param([gcb '/Integer Delay'],'NumDelays',num2str(Delay));
      |     set_param([gcb '/Delay'],'Value',num2str(Delay));
      | end
      mask Display: text(0.5,0.5,['z^{ ' num2str((-1)*str2double(get_param(gcb,'Delay'))) '}'],'texmode','on');
  EUL delay : Subsystem  TreatAsAtomicUnit=on  mask{Delay=0}
      mask prompts: Delay "Delay (in simulation steps) for the input signal:"
      mask init:
      | %set_param([gcb '/Discrete Transfer Fcn'],'Denominator',['[' num2str([1 zeros(1,str2double(get_param(gcb,'Delay')))]) ']']);
      mask CallbackString:
      | Delay = str2double(get_param(gcb,'Delay'));
      | if Delay < 0
      |     set_param(gcb,'Delay','0');
      |     error('Only non-negative delays are possible (causality).');
      |     set_param([gcb '/Delay'],'Value','0');
      | elseif Delay == 0
      |     set_param([gcb '/Delay'],'Value','0');
      | else
      |     set_param([gcb '/Integer Delay'],'NumDelays',num2str(Delay));
      |     set_param([gcb '/Delay'],'Value',num2str(Delay));
      | end
      mask Display: text(0.5,0.5,['z^{ ' num2str((-1)*str2double(get_param(gcb,'Delay'))) '}'],'texmode','on');
  ELLout : Outport  OutDataType=sfix(16)  OutScaling=2^0
  EULout : Outport  Port=2  OutDataType=sfix(16)  OutScaling=2^0
  ADout : Outport  Port=3  OutDataType=sfix(16)  OutScaling=2^0
  wires:
  ELLin/1 -> ELL delay/1(In1)
  EULin/1 -> EUL delay/1(In1)
  ADin/1 -> AD delay/1(In1)
  ELL delay/1(Out1) -> ELLout/1
  EUL delay/1(Out1) -> EULout/1
  AD delay/1(Out1) -> ADout/1

== system Pedal_Interpretation_exe/Validation Functions/SR-PI-01.1 Brake Pedal recognition/BrakePedal == 0/PAS/Ra delay ==
  In1 : Inport  OutDataType=sfix(16)  OutScaling=2^0
  Data Type Conversion : DataTypeConversion  OutDataType=sfix(16)  OutScaling=2^0
  Delay : Constant  Value=0  OutDataType=sfix(16)  OutScaling=2^0
  Integer Delay : S-Function  FunctionName=sfix_udelay  Parameters=samptime,vinit,NumDelays,1,1,0  mask(Integer Delay){vinit=0.0, samptime=-1, NumDelays=15}
      mask prompts: vinit "Initial condition:"; samptime "Sample time:"; NumDelays "Number of delays:"
      mask help: Delay a signal N sample periods.
      mask init:
      | if isempty(NumDelays)
      |    NumDelays = 1;
      | end
      mask Display: fprintf(' %d\nZ   ',-1*(NumDelays))
  Switch : Switch  Criteria=u2 ~= 0
  Out1 : Outport  OutDataType=sfix(16)  OutScaling=2^0
  wires:
  Data Type Conversion/1 -> Out1/1
  Integer Delay/1 -> Switch/1
  Delay/1 -> Switch/2
  In1/1 -> Integer Delay/1, Switch/3
  Switch/1 -> Data Type Conversion/1

== system Pedal_Interpretation_exe/Validation Functions/SR-PI-01.1 Brake Pedal recognition/BrakePedal == 0/PAS/Rp delay ==
  In1 : Inport  OutDataType=sfix(16)  OutScaling=2^0
  Data Type Conversion : DataTypeConversion  OutDataType=sfix(16)  OutScaling=2^0
  Delay : Constant  Value=0  OutDataType=sfix(16)  OutScaling=2^0
  Integer Delay : S-Function  FunctionName=sfix_udelay  Parameters=samptime,vinit,NumDelays,1,1,0  mask(Integer Delay){vinit=0.0, samptime=-1, NumDelays=600}
      mask prompts: vinit "Initial condition:"; samptime "Sample time:"; NumDelays "Number of delays:"
      mask help: Delay a signal N sample periods.
      mask init:
      | if isempty(NumDelays)
      |    NumDelays = 1;
      | end
      mask Display: fprintf(' %d\nZ   ',-1*(NumDelays))
  Switch : Switch  Criteria=u2 ~= 0
  Out1 : Outport  OutDataType=sfix(16)  OutScaling=2^0
  wires:
  Data Type Conversion/1 -> Out1/1
  Integer Delay/1 -> Switch/1
  Delay/1 -> Switch/2
  In1/1 -> Integer Delay/1, Switch/3
  Switch/1 -> Data Type Conversion/1

== system Pedal_Interpretation_exe/Validation Functions/SR-PI-01.1 Brake Pedal recognition/BrakePedal == 0/PAS/Ta delay ==
  In1 : Inport  OutDataType=sfix(16)  OutScaling=2^0
  Data Type Conversion : DataTypeConversion  OutDataType=sfix(16)  OutScaling=2^0
  Delay : Constant  Value=0  OutDataType=sfix(16)  OutScaling=2^0
  Integer Delay : S-Function  FunctionName=sfix_udelay  Parameters=samptime,vinit,NumDelays,1,1,0  mask(Integer Delay){vinit=0.0, samptime=-1, NumDelays=15}
      mask prompts: vinit "Initial condition:"; samptime "Sample time:"; NumDelays "Number of delays:"
      mask help: Delay a signal N sample periods.
      mask init:
      | if isempty(NumDelays)
      |    NumDelays = 1;
      | end
      mask Display: fprintf(' %d\nZ   ',-1*(NumDelays))
  Switch : Switch  Criteria=u2 ~= 0
  Out1 : Outport  OutDataType=sfix(16)  OutScaling=2^0
  wires:
  Data Type Conversion/1 -> Out1/1
  Integer Delay/1 -> Switch/1
  Delay/1 -> Switch/2
  In1/1 -> Integer Delay/1, Switch/3
  Switch/1 -> Data Type Conversion/1

== system Pedal_Interpretation_exe/Validation Functions/SR-PI-01.1 Brake Pedal recognition/BrakePedal == 0/PAS/Tp delay ==
  In1 : Inport  OutDataType=sfix(16)  OutScaling=2^0
  Data Type Conversion : DataTypeConversion  OutDataType=sfix(16)  OutScaling=2^0
  Delay : Constant  Value=0  OutDataType=sfix(16)  OutScaling=2^0
  Integer Delay : S-Function  FunctionName=sfix_udelay  Parameters=samptime,vinit,NumDelays,1,1,0  mask(Integer Delay){vinit=0.0, samptime=-1, NumDelays=600}
      mask prompts: vinit "Initial condition:"; samptime "Sample time:"; NumDelays "Number of delays:"
      mask help: Delay a signal N sample periods.
      mask init:
      | if isempty(NumDelays)
      |    NumDelays = 1;
      | end
      mask Display: fprintf(' %d\nZ   ',-1*(NumDelays))
  Switch : Switch  Criteria=u2 ~= 0
  Out1 : Outport  OutDataType=sfix(16)  OutScaling=2^0
  wires:
  Data Type Conversion/1 -> Out1/1
  Integer Delay/1 -> Switch/1
  Delay/1 -> Switch/2
  In1/1 -> Integer Delay/1, Switch/3
  Switch/1 -> Data Type Conversion/1

== system Pedal_Interpretation_exe/Validation Functions/SR-PI-01.1 Brake Pedal recognition/BrakePedal == 0/PAS/V delay ==
  In1 : Inport  OutDataType=sfix(16)  OutScaling=2^0
  Data Type Conversion : DataTypeConversion  OutDataType=sfix(16)  OutScaling=2^0
  Delay : Constant  Value=0  OutDataType=sfix(16)  OutScaling=2^0
  Integer Delay : S-Function  FunctionName=sfix_udelay  Parameters=samptime,vinit,NumDelays,1,1,0  mask(Integer Delay){vinit=0.0, samptime=-1, NumDelays=15}
      mask prompts: vinit "Initial condition:"; samptime "Sample time:"; NumDelays "Number of delays:"
      mask help: Delay a signal N sample periods.
      mask init:
      | if isempty(NumDelays)
      |    NumDelays = 1;
      | end
      mask Display: fprintf(' %d\nZ   ',-1*(NumDelays))
  Switch : Switch  Criteria=u2 ~= 0
  Out1 : Outport  OutDataType=sfix(16)  OutScaling=2^0
  wires:
  Data Type Conversion/1 -> Out1/1
  Integer Delay/1 -> Switch/1
  Delay/1 -> Switch/2
  In1/1 -> Integer Delay/1, Switch/3
  Switch/1 -> Data Type Conversion/1

== system Pedal_Interpretation_exe/Validation Functions/SR-PI-01.1 Brake Pedal recognition/BrakePedal == 0/PAS/error ==
  Rp : Inport  OutDataType=sfix(16)  OutScaling=2^0
  Tp : Inport  Port=2  OutDataType=sfix(16)  OutScaling=2^0
  A : Inport  Port=3  OutDataType=sfix(16)  OutScaling=2^0
  Ra : Inport  Port=4  OutDataType=sfix(16)  OutScaling=2^0
  Ta : Inport  Port=5  OutDataType=sfix(16)  OutScaling=2^0
  V : Inport  Port=6  OutDataType=sfix(16)  OutScaling=2^0
  Compare To Constant{,2,4,6,8,10} (6 alike) : simulink/Logic and Bit Operations/Compare To Constant  SystemSampleTime=-1  relop===  const=0  LogicOutDataTypeMode=uint8  ZeroCross=off
  Compare To Constant{1,3,5,7,9,11} (6 alike) : simulink/Logic and Bit Operations/Compare To Constant  SystemSampleTime=-1  relop===  const=1  LogicOutDataTypeMode=uint8  ZeroCross=off
  Logical Operator{,1,3..6} (6 alike) : Logic  Operator=NOR  AllPortsSameDT=off  OutDataTypeMode=boolean
  Logical Operator2 : Logic  Operator=OR  Inputs=6  AllPortsSameDT=off  OutDataTypeMode=boolean
  Verror : Outport  OutDataType=sfix(16)  OutScaling=2^0
  wires:
  Logical Operator6/1 -> Logical Operator2/6
  Logical Operator5/1 -> Logical Operator2/5
  Logical Operator4/1 -> Logical Operator2/4
  Logical Operator3/1 -> Logical Operator2/3
  Logical Operator1/1 -> Logical Operator2/2
  Logical Operator/1 -> Logical Operator2/1
  V/1 -> Compare To Constant11/1, Compare To Constant10/1
  Compare To Constant10/1 -> Logical Operator6/1
  Compare To Constant11/1 -> Logical Operator6/2
  A/1 -> Compare To Constant5/1, Compare To Constant4/1
  Compare To Constant4/1 -> Logical Operator3/1
  Compare To Constant5/1 -> Logical Operator3/2
  Compare To Constant/1 -> Logical Operator/1
  Compare To Constant1/1 -> Logical Operator/2
  Compare To Constant2/1 -> Logical Operator1/1
  Compare To Constant3/1 -> Logical Operator1/2
  Logical Operator2/1 -> Verror/1
  Rp/1 -> Compare To Constant/1, Compare To Constant1/1
  Tp/1 -> Compare To Constant2/1, Compare To Constant3/1
  Ra/1 -> Compare To Constant6/1, Compare To Constant7/1
  Compare To Constant6/1 -> Logical Operator4/1
  Compare To Constant7/1 -> Logical Operator4/2
  Ta/1 -> Compare To Constant9/1, Compare To Constant8/1
  Compare To Constant8/1 -> Logical Operator5/1
  Compare To Constant9/1 -> Logical Operator5/2
